simulink model "testAlphaWindowOut"  (R2018b)
settings: Solver=VariableStepDiscrete  StartTime=12*3600  StopTime=20+12*3600  MaxStep=0.4  RelTol=1e-3  EnableMultiTasking=on
libraries: carnot x5, simulink x1
settings Model: Creator=drhf  LastModifiedBy=drhf
settings DataIOCC: LimitDataPoints=on  SaveFormat=Array  ReturnWorkspaceOutputs=on
settings OptimizationCC: DefaultParameterBehavior=Inlined  LifeSpan=inf
settings DebuggingCC: ReadBeforeWriteMsg=DisableAll  WriteAfterWriteMsg=DisableAll  WriteAfterReadMsg=DisableAll  UnderspecifiedInitializationDetection=Classic  MergeDetectMultiDrivingBlocksExec=none  SolverPrmCheckMsg=warning  MultiTaskDSMMsg=none  SFUnexpectedBacktrackingDiag=warning  SFNoUnconditionalDefaultTransitionDiag=warning  SFExecutionAtInitializationDiag=none
settings HardwareCC: ProdBitPerPointer=32  ProdBitPerSizeT=32  ProdBitPerPtrDiffT=32  ProdLargestAtomicFloat=None  ProdIntDivRoundTo=Undefined  ProdEndianess=Unspecified  ProdWordSize=32  ProdHWDeviceType=32-bit Generic
settings ModelReferenceCC: UpdateModelReferenceTargets=IfOutOfDate  PropagateSignalLabelsOutOfModel=off
settings SFSimCC: SFSimEcho=off  SimUseLocalCustomCode=off
settings RTWCC: RTWUseLocalCustomCode=off
settings CodeAppCC: StateflowObjectComments=on
settings GRTTargetCC: TargetLangStandard=C89/C90 (ANSI)  GeneratePreprocessorConditionals=Disable all
settings ConfigComp: CovMetricSettings=dw  CovHtmlReporting=on  CovSaveCumulativeToWorkspaceVar=on  CovSaveSingleToWorkspaceVar=on  CovExternalEMLEnable=off

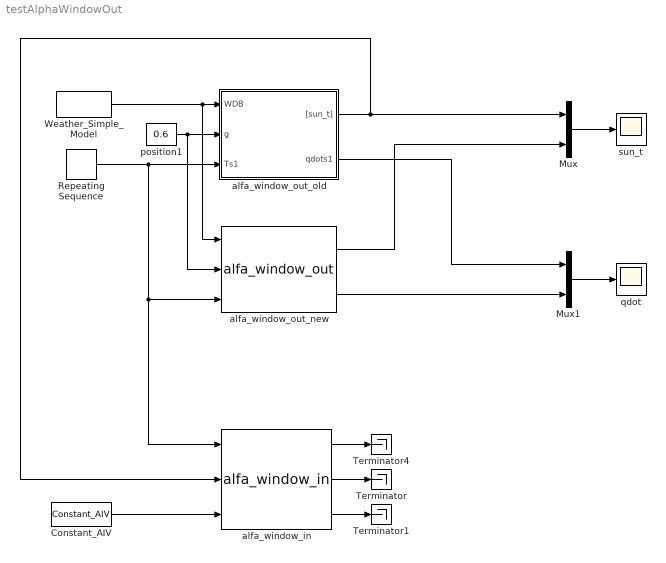
== system testAlphaWindowOut ==
  Constant_AIV : carnot/Source/Ventilation/Constant_AIV  Tsens=20  Tcon=20  Trad=20  mw=0.012  mco=0.01  rhoair=1.2  cpair=1004  pair=100000  nair=0.5
  Mux : Mux  Inputs=2
  Mux1 : Mux  Inputs=2
  Repeating Sequence : simulink/Sources/Repeating Sequence  rep_seq_t=[0 10]  rep_seq_y=[10 30]
  Terminator : Terminator
  Terminator1 : Terminator
  Terminator4 : Terminator
  Weather_Simple_Model : carnot/Weather/Weather_Simple_Model  lat=60  Ibn=900  Idg=100  tamb=5  deltaTsky=-6  rh=50  precip="10e-3/24/3600           % 10 mm in 24 h"  cloud=0.125  p=1013e2  vw=1  wdir=270
  alfa_window_in : carnot/Basic/Heat_Transfer/alfa_window_in  gvalue=0.7  emission_in=0.87  wallsurface=1  frame=0.1  numlayer=2
  alfa_window_out_new : carnot/Basic/Heat_Transfer/alfa_window_out  pos=0  absorption_out=0.01  emission_out=0.87  frame=0.1
  alfa_window_out_old : Subsystem  mask(ALFA){pos=0, absorption_out=0.01, emission_out=0.87, frame=0.1}
      mask prompts: pos "Azimut of the surface (South = 0; East = -90)"; absorption_out "Solar absorption of the glass (0...1)"; emission_out "Longwave emissivity (0...1)"; frame "Share of the frame on the surface (0..1)"
      mask help:
      | Convective and radiative heat transfer at the OUTDOOR SURFACE OF A VERTICAL WINDOW.
      | Azimut can be a scalar or a vector with [inclination azimut rotation].
      | [W*] : modified weather data, adapted to height over ground,
      | Ts : temperature of outdoor window surface, °C,
      | qdots : specific heat flow into window construction, W/m^2,
      | [sun_t] : sun data (incidence angle, direct and diffuse radiation
      |                  at tilted window surface).
      mask init:
      | if length(pos) == 1
      |     pos = [90  pos 0]; % pos is [inclination azimut rotation]
      | end
  position1 : Constant  Value=0.6
  qdot : Scope
  sun_t : Scope
  wires:
  Repeating Sequence/1 -> alfa_window_out_old/3(Ts1), alfa_window_out_new/3, alfa_window_in/1
  Mux/1 -> sun_t/1
  Weather_Simple_Model/1 -> alfa_window_out_new/1, alfa_window_out_old/1(WDB)
  Constant_AIV/1 -> alfa_window_in/3
  position1/1 -> alfa_window_out_new/2, alfa_window_out_old/2(g)
  alfa_window_out_old/1("[sun_t]") -> alfa_window_in/2, Mux/1
  alfa_window_in/2 -> Terminator/1
  alfa_window_in/3 -> Terminator1/1
  alfa_window_in/1 -> Terminator4/1
  Mux1/1 -> qdot/1
  alfa_window_out_old/2(qdots1) -> Mux1/1
  alfa_window_out_new/1 -> Mux/2
  alfa_window_out_new/2 -> Mux1/2

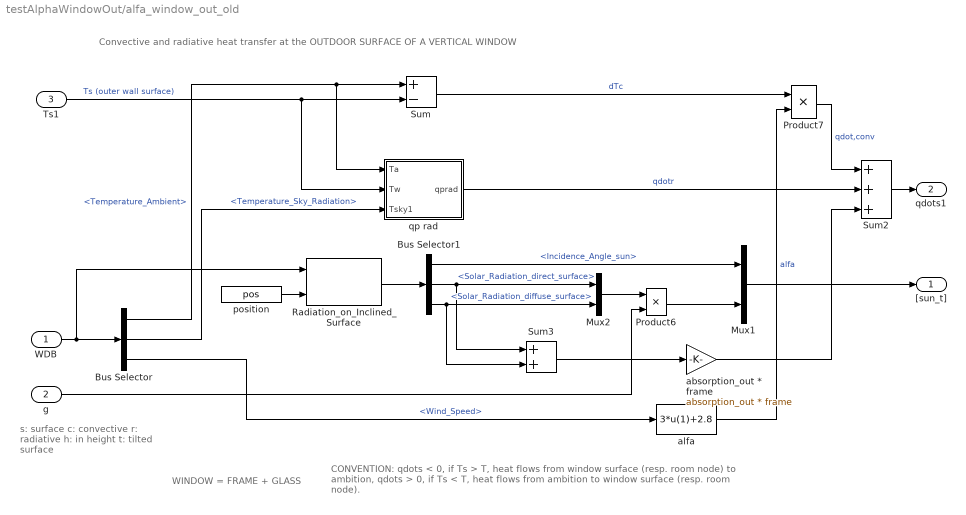
== system testAlphaWindowOut/alfa_window_out_old ==
  note: CONVENTION:
      | qdots < 0, if Ts > T, heat flows from window surface (resp. room node) to ambition,
      | qdots > 0, if Ts < T, heat flows from ambition to window surface (resp. room node).
  note: s: surface
      | c: convective
      | r: radiative
      | h: in height
      | t: tilted surface
  note: Convective and radiative heat transfer at the OUTDOOR SURFACE OF A VERTICAL WINDOW
  note: WINDOW = FRAME + GLASS
  WDB : Inport
  g : Inport  Port=2
  Ts1 : Inport  Port=3
  Bus Selector : BusSelector  OutputSignals=Temperature_Ambient,Temperature_Sky_Radiation,Wind_Speed
  Bus Selector1 : BusSelector  OutputSignals=Incidence_Angle_sun,Solar_Radiation_direct_surface,Solar_Radiation_diffuse_surface
  Mux1 : Mux  Inputs=2
  Mux2 : Mux  Inputs=2
  Product6 : Product  SaturateOnIntegerOverflow=on  InputSameDT=on  OutDataTypeStr=Inherit: Same as first input
  Product7 : Product  SaturateOnIntegerOverflow=on  InputSameDT=on  OutDataTypeStr=Inherit: Same as first input
  Radiation_on_Inclined_Surface : carnot/Weather/Radiation_on_Inclined_Surface  sky=Perez 1990  reflect=0.2
  Sum : Sum  Inputs=+-  SaturateOnIntegerOverflow=on  InputSameDT=on  OutDataTypeStr=Inherit: Same as first input
  Sum2 : Sum  Inputs=+++  SaturateOnIntegerOverflow=on  InputSameDT=on  OutDataTypeStr=Inherit: Same as first input
  Sum3 : Sum  SaturateOnIntegerOverflow=on  InputSameDT=on  OutDataTypeStr=Inherit: Same as first input
  absorption_out * frame : Gain  Gain=absorption_out * frame  SaturateOnIntegerOverflow=on  OutDataTypeStr=Inherit: Same as input  ParamDataTypeStr=Inherit: Same as input
  alfa : Fcn  Expr=3*u(1)+2.8
  position : Constant  Value=pos
  qp rad : Subsystem
  "[sun_t]" : Outport
  qdots1 : Outport  Port=2
  wires:
  Bus Selector/3 -> alfa/1  "<Wind_Speed>"
  Bus Selector/2 -> qp rad/3(Tsky1)  "<Temperature_Sky_Radiation>"
  Bus Selector/1 -> Sum/1, qp rad/1(Ta)  "<Temperature_Ambient>"
  Bus Selector1/3 -> Sum3/2, Mux2/2  "<Solar_Radiation_diffuse_surface>"
  Mux2/1 -> Product6/1
  Product6/1 -> Mux1/2
  Sum/1 -> Product7/1  "dTc"
  WDB/1 -> Bus Selector/1, Radiation_on_Inclined_Surface/1
  Bus Selector1/1 -> Mux1/1  "<Incidence_Angle_sun>"
  Sum3/1 -> absorption_out * frame/1
  Sum2/1 -> qdots1/1
  g/1 -> Product6/2
  absorption_out * frame/1 -> Sum2/3
  Bus Selector1/2 -> Sum3/1, Mux2/1  "<Solar_Radiation_direct_surface>"
  Mux1/1 -> "[sun_t]"/1
  Ts1/1 -> Sum/2, qp rad/2(Tw)  "Ts (outer wall surface)"
  qp rad/1(qprad) -> Sum2/2  "qdotr"
  alfa/1 -> Product7/2  "alfa"
  Product7/1 -> Sum2/1  "qdot,conv"
  position/1 -> Radiation_on_Inclined_Surface/2
  Radiation_on_Inclined_Surface/1 -> Bus Selector1/1

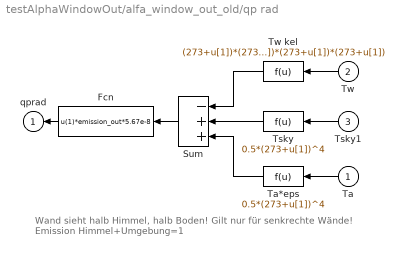
== system testAlphaWindowOut/alfa_window_out_old/qp rad ==
  note: Wand sieht halb Himmel, halb Boden! Gilt nur für senkrechte Wände!
      | Emission Himmel+Umgebung=1
  Ta : Inport
  Tw : Inport  Port=2
  Tsky1 : Inport  Port=3
  Fcn : Fcn  Expr=u(1)*emission_out*5.67e-8
  Sum : Sum  Inputs=-++  SaturateOnIntegerOverflow=on  InputSameDT=on  OutDataTypeStr=Inherit: Same as first input
  Ta*eps : Fcn  Expr=0.5*(273+u[1])^4
  Tsky : Fcn  Expr=0.5*(273+u[1])^4
  Tw kel : Fcn  Expr=(273+u[1])*(273+u[1])*(273+u[1])*(273+u[1])
  qprad : Outport
  wires:
  Tsky/1 -> Sum/2
  Tw kel/1 -> Sum/1
  Tw/1 -> Tw kel/1
  Ta*eps/1 -> Sum/3
  Sum/1 -> Fcn/1
  Fcn/1 -> qprad/1
  Ta/1 -> Ta*eps/1
  Tsky1/1 -> Tsky/1
